simulink model "Exercice2_Simulink_Lise_TUONG_2PH2"  (R2025b)
settings: Solver=VariableStepAuto  StartTime=0.0  StopTime=4  RelTol=1e-3
model workspace (MAT data in the model file):
  a = 1
undefined symbols (not defined in the file): C, R
libraries: simulink x1
settings Model: Creator=liset  LastModifiedBy=liset

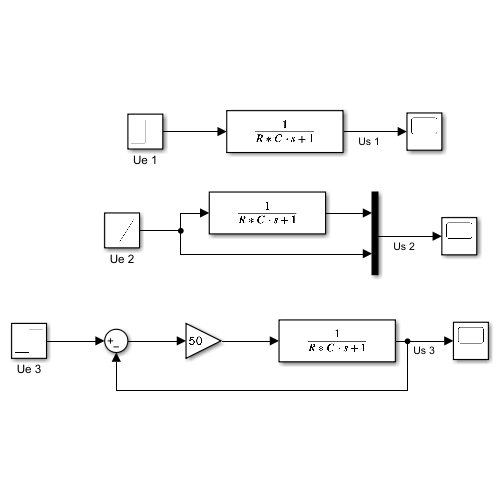
[thumbnail: Simulink's stored preview of the top-level diagram]
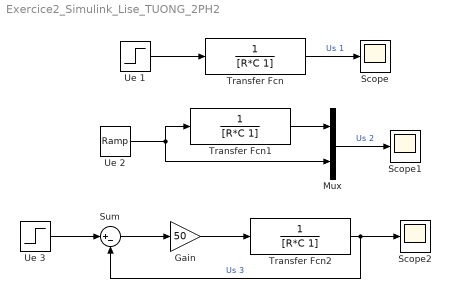
== system Exercice2_Simulink_Lise_TUONG_2PH2 ==
  Gain : Gain  Gain=50
  Mux : Mux  Inputs=2
  Scope : Scope
      settings: ActiveDisplayYMinimum=-0.12495806717134714  ActiveDisplayYMaximum=1.1246226045421244
  Scope1 : Scope
      settings: ActiveDisplayYMinimum=-0.49999999999999989  ActiveDisplayYMaximum=4.5
  Scope2 : Scope
      settings: ActiveDisplayYMinimum=-0.12253930611943123  ActiveDisplayYMaximum=1.1028537550748814  DataLoggingVariableName=ScopeData2
  Sum : Sum  Inputs=|+-
  Transfer Fcn : TransferFcn  Denominator=[R*C 1]
  Transfer Fcn1 : TransferFcn  Denominator=[R*C 1]
  Transfer Fcn2 : TransferFcn  Denominator=[R*C 1]
  Ue 1 : Step  Time=0  SampleTime=0
  Ue 2 : simulink/Sources/Ramp  slope=1  start=0  InitialOutput=0
  Ue 3 : Step  Time=0  SampleTime=0
  wires:
  Sum/1 -> Gain/1
  Mux/1 -> Scope1/1  "Us 2"
  Transfer Fcn1/1 -> Mux/1
  Ue 2/1 -> Mux/2, Transfer Fcn1/1
  Gain/1 -> Transfer Fcn2/1
  Transfer Fcn2/1 -> Scope2/1, Sum/2  "Us 3"
  Ue 1/1 -> Transfer Fcn/1
  Ue 3/1 -> Sum/1
  Transfer Fcn/1 -> Scope/1  "Us 1"
